simulink model "controller"  (R2015a)
settings: Solver=ode45  StartTime=0.0  StopTime=10.0  RelTol=1e-3
libraries: fuzblock x2
settings Model: Creator=BML  LastModifiedBy=BML

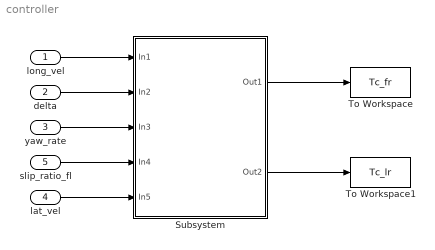
== system controller ==
  "  long_vel  " : Inport
  "  delta " : Inport  Port=2
  "  yaw_rate " : Inport  Port=3
  "  lat_vel" : Inport  Port=4
  " slip_ratio_fl  " : Inport  Port=5
  Subsystem : Subsystem
  To Workspace : ToWorkspace  VariableName=Tc_fr  SaveFormat=Timeseries  SampleTime=-1
  To Workspace1 : ToWorkspace  VariableName=Tc_lr  SaveFormat=Timeseries  SampleTime=-1
  wires:
  "  long_vel  "/1 -> Subsystem/1(In1)
  "  delta "/1 -> Subsystem/2(In2)
  "  yaw_rate "/1 -> Subsystem/3(In3)
  " slip_ratio_fl  "/1 -> Subsystem/4(In4)
  "  lat_vel"/1 -> Subsystem/5(In5)
  Subsystem/1(Out1) -> To Workspace/1
  Subsystem/2(Out2) -> To Workspace1/1

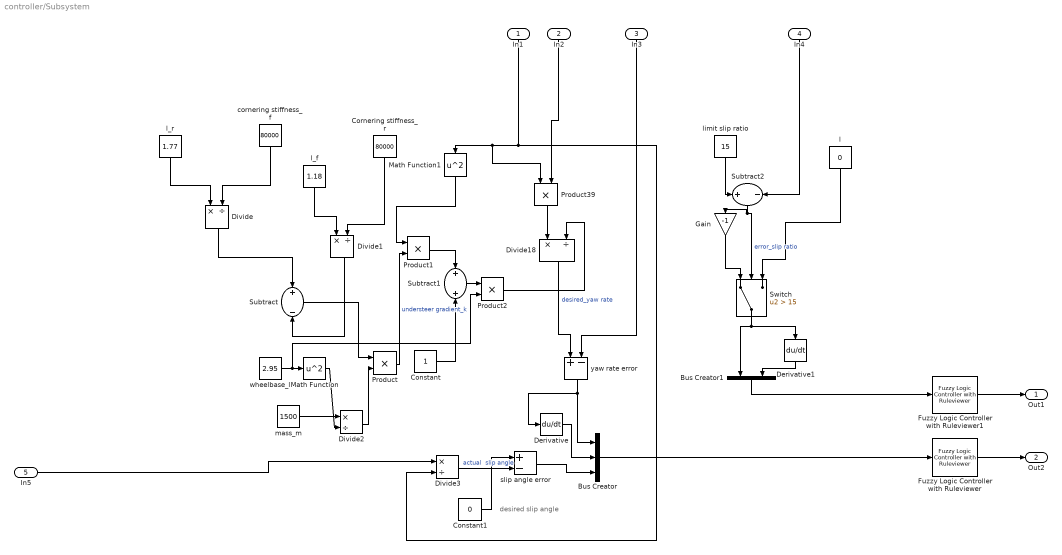
== system controller/Subsystem ==
  note: desired
      | slip angle
  In1 : Inport
  In2 : Inport  Port=2
  In3 : Inport  Port=3
  In4 : Inport  Port=4
  In5 : Inport  Port=5
  Bus Creator : BusCreator  Inputs=3
  Bus Creator1 : BusCreator  Inputs=2
  Constant : Constant
  Constant1 : Constant  Value=0
  "Cornering stiffness_r " : Constant  Value=80000
  Derivative : Derivative
  Derivative1 : Derivative
  Divide{,1..3,18} (5 alike) : Product  Inputs=*/
  Fuzzy Logic Controller with Ruleviewer : fuzblock/Fuzzy Logic  Controller  with Ruleviewer  fismatrix=yaw_rate  Ts=2
  Fuzzy Logic Controller with Ruleviewer1 : fuzblock/Fuzzy Logic  Controller  with Ruleviewer  fismatrix=slip_ratio  Ts=2
  Gain : Gain  Gain=-1
  Math Function : Math  Operator=square  SaturateOnIntegerOverflow=on
  Math Function1 : Math  Operator=square  SaturateOnIntegerOverflow=on
  Product{,1..2,39} (4 alike) : Product
  Subtract : Sum  Inputs=+-
  Subtract1 : Sum
  Subtract2 : Sum  Inputs=+-
  Switch : Switch  Criteria=u2 > Threshold  Threshold=15
  "cornering stiffness_f " : Constant  Value=80000
  l : Constant  Value=0
  "l_f " : Constant  Value=1.18
  "l_r " : Constant  Value=1.77
  limit slip ratio : Constant  Value=15
  mass_m : Constant  Value=1500
  "slip angle error  " : Sum  Inputs=+-
  wheelbase_l : Constant  Value=2.95
  "yaw rate error   " : Sum  Inputs=+-
  Out1 : Outport
  Out2 : Outport  Port=2
  wires:
  Fuzzy Logic Controller with Ruleviewer1/1 -> Out1/1
  Divide/1 -> Subtract/1
  Subtract/1 -> Product/1
  Product/1 -> Product1/2  "understeer gradient_k"
  Constant/1 -> Subtract1/2
  Product39/1 -> Divide18/1
  Product2/1 -> Divide18/2
  In2/1 -> Product39/2
  Math Function1/1 -> Product1/1
  Subtract1/1 -> Product2/1
  In5/1 -> Divide3/1
  "l_r "/1 -> Divide/1
  Divide1/1 -> Subtract/2
  "Cornering stiffness_r "/1 -> Divide1/2
  wheelbase_l/1 -> Product2/2, Math Function/1
  mass_m/1 -> Divide2/1
  Math Function/1 -> Divide2/2
  Divide2/1 -> Product/2
  In1/1 -> Divide3/2, Math Function1/1, Product39/1
  "l_f "/1 -> Divide1/1
  "cornering stiffness_f "/1 -> Divide/2
  Product1/1 -> Subtract1/1
  Constant1/1 -> "slip angle error  "/1
  Switch/1 -> Derivative1/1, Bus Creator1/1
  In3/1 -> "yaw rate error   "/2
  Divide18/1 -> "yaw rate error   "/1  "desired_yaw rate"
  Subtract2/1 -> Switch/2, Gain/1  "error_slip ratio"
  Gain/1 -> Switch/1
  "yaw rate error   "/1 -> Bus Creator/1, Derivative/1
  limit slip ratio/1 -> Subtract2/1
  Derivative/1 -> Bus Creator/2
  Bus Creator/1 -> Fuzzy Logic Controller with Ruleviewer/1
  In4/1 -> Subtract2/2
  l/1 -> Switch/3
  Divide3/1 -> "slip angle error  "/2  "actual  slip angle"
  "slip angle error  "/1 -> Bus Creator/3
  Derivative1/1 -> Bus Creator1/2
  Bus Creator1/1 -> Fuzzy Logic Controller with Ruleviewer1/1
  Fuzzy Logic Controller with Ruleviewer/1 -> Out2/1
